simulink library "carnotUIBK"  (R2024b)
settings: Solver=VariableStepAuto  StartTime=0.0  StopTime=10.0  RelTol=1e-3  EnableMultiTasking=on
values from neighbouring files (symbols this model uses):
  area = area + room(kk).area    [THERMALZONE.m]
  boundary = BOUNDARY()    [BUILDING.m]
  building = obj    [BUILDING.m]
  C = zeros(1,length(d)+1)    [CONSTRUCTION.m]
  cp = str2num(value)    [CONSTRUCTION.m]
  pos = find(d_layer>0)    [CONSTRUCTION.m]
  rho = str2num(value)    [CONSTRUCTION.m]
  type = 1    [CONSTRUCTION.m]
  zone = obj.zone(ind)    [THERMALZONE.m]
undefined symbols (not defined in the file or in its folder): A, amb_factor, B, const, control, Dd, get_building, height, p, Qdot_C, Qdot_H, Qdot_I_electricity, Qdot_I_light, Qdot_I_person, Qdot_S, Qdot_T_ground, Qdot_T_neighbour, Qdot_T_opaque, Qdot_T_window, Qdot_V_infiltration, Qdot_V_mech, Qdot_V_window, r_frame, solar_ratio, solar_ratio1, solar_ratio2, Tc, Tr, Ts, Uvalue, view_factor, wall, wallsurface, window, window_height, window_heigth, window_width, windowsurface, x_CO2, x_H2O, x_VOC, z
libraries: carnot x105, $bdroot x22, simulink x18, simulink_extras x14
(part 9 of 13)

== system carnotUIBK/gain/People/W//ppl (activity)/LUT_Qdot_hum1 ==
  note: LATENT/HUMID HEAT POWER emitted from a person in a room
  activity : Inport
  Top : Inport  Port=2
  Look-Up Table Qdot_hum : Subsystem  mask(Lookup Table (2-D)){x=[10 12 14 16 18 20 22 23 24 25 26 28 30 32 34], y=[0 1 2 3 4], t=[20 20 20 55 100; 20 20 20 55 100; 20 20 20 55 100; 21 21 21 58 105; 23 23 23 65 115; 25 25 25 75 130; 30 30 30 85 145; 35 35 35 90 155; 40 40 40 95 160; 45 45 45 100 167; 50 50 50 105 175; 60 60 60 115 190; 70 70 70 125 205; 80 80 80 135 225; 90 90 90 145 245]}
      mask prompts: x "Row:"; y "Column:"; t "Table:"
      mask help: Performs 2-D linear interpolation of input values using the specified input/output table. Extrapolation is performed outside the table boundaries.
      mask init:
      | [r,c]=size(t);
      | x=reshape(x,prod(size(x)),1);
      | xi=x(:,ones(1,c));
      | minx=min(x); maxx=max(x);
      | mint=min(min(t)); maxt=max(max(t));
      mask Display: plot(xi,t,[minx maxx],[mint mint],[minx minx],[mint maxt])
  Qdot_hum : Outport  InitialOutput=0  VectorParamsAs1DForOutWhenUnconnected=off
  wires:
  Top/1 -> Look-Up Table Qdot_hum/1(Rows)
  activity/1 -> Look-Up Table Qdot_hum/2(Cols)
  Look-Up Table Qdot_hum/1(U) -> Qdot_hum/1

== system carnotUIBK/gain/People/W//ppl (activity)/LUT_mdot_CO2 ==
  note: CO2 MASS FLOW emitted from a person in a room
  activity : Inport
  Look-Up mdot_CO2 : Lookup  InputValues=[0 1 2 3 4]  Table=[0.567 0.708 1.133 2.031 3.305]*10^-5
  mdot_CO2 : Outport  InitialOutput=0  VectorParamsAs1DForOutWhenUnconnected=off
  wires:
  Look-Up mdot_CO2/1 -> mdot_CO2/1
  activity/1 -> Look-Up mdot_CO2/1

== system carnotUIBK/gain/People/W//ppl (activity)/LUT_mdot_H2O ==
  note: WATER MASS FLOW emitted from a person in a room
  activity : Inport
  Top : Inport  Port=2
  Look-Up Table mdot_H2O : Subsystem  mask(Lookup Table (2-D)){x=[10 12 14 16 18 20 22 23 24 25 26 32], y=[0 1 2 3 4], t=[30 30 30 90 150; 30 30 30 90 150; 30 30 30 90 150; 30 30 30 90 155; 35 35 35 95 165; 40 40 40 110 185; 45 45 45 125 200; 50 50 50 130 210; 55 55 55 130 225; 60 60 60 140 240; 65 65 65 150 270; 120 120 120 250 450]/(3.6*1e6)}
      mask prompts: x "Row:"; y "Column:"; t "Table:"
      mask help: Performs 2-D linear interpolation of input values using the specified input/output table. Extrapolation is performed outside the table boundaries.
      mask init:
      | [r,c]=size(t);
      | x=reshape(x,prod(size(x)),1);
      | xi=x(:,ones(1,c));
      | minx=min(x); maxx=max(x);
      | mint=min(min(t)); maxt=max(max(t));
      mask Display: plot(xi,t,[minx maxx],[mint mint],[minx minx],[mint maxt])
  mdot_H2O : Outport  InitialOutput=0  VectorParamsAs1DForOutWhenUnconnected=off
  wires:
  Look-Up Table mdot_H2O/1(U) -> mdot_H2O/1
  activity/1 -> Look-Up Table mdot_H2O/2(Cols)
  Top/1 -> Look-Up Table mdot_H2O/1(Rows)

== system carnotUIBK/gain/People/W//ppl (constant)/LUT_mdot_CO2 ==
  note: CO2 MASS FLOW emitted from a person in a room
  activity : Inport
  Look-Up mdot_CO2 : Lookup  InputValues=[0 1 2 3 4]  Table=[0.567 0.708 1.133 2.031 3.305]*10^-5
  mdot_CO2 : Outport  InitialOutput=0  VectorParamsAs1DForOutWhenUnconnected=off
  wires:
  Look-Up mdot_CO2/1 -> mdot_CO2/1
  activity/1 -> Look-Up mdot_CO2/1

== system carnotUIBK/gain/People/W//ppl (constant)/LUT_mdot_H2O ==
  note: WATER MASS FLOW emitted from a person in a room
  activity : Inport
  Top : Inport  Port=2
  Look-Up Table mdot_H2O : Subsystem  mask(Lookup Table (2-D)){x=[10 12 14 16 18 20 22 23 24 25 26 32], y=[0 1 2 3 4], t=[30 30 30 90 150; 30 30 30 90 150; 30 30 30 90 150; 30 30 30 90 155; 35 35 35 95 165; 40 40 40 110 185; 45 45 45 125 200; 50 50 50 130 210; 55 55 55 130 225; 60 60 60 140 240; 65 65 65 150 270; 120 120 120 250 450]/(3.6*1e6)}
      mask prompts: x "Row:"; y "Column:"; t "Table:"
      mask help: Performs 2-D linear interpolation of input values using the specified input/output table. Extrapolation is performed outside the table boundaries.
      mask init:
      | [r,c]=size(t);
      | x=reshape(x,prod(size(x)),1);
      | xi=x(:,ones(1,c));
      | minx=min(x); maxx=max(x);
      | mint=min(min(t)); maxt=max(max(t));
      mask Display: plot(xi,t,[minx maxx],[mint mint],[minx minx],[mint maxt])
  mdot_H2O : Outport  InitialOutput=0  VectorParamsAs1DForOutWhenUnconnected=off
  wires:
  Look-Up Table mdot_H2O/1(U) -> mdot_H2O/1
  activity/1 -> Look-Up Table mdot_H2O/2(Cols)
  Top/1 -> Look-Up Table mdot_H2O/1(Rows)

== system carnotUIBK/infiltration/infiltration_pressure/infiltration_pressure/dP_infiltration ==
  T_int : Inport
  T_ext : Inport  Port=2
  windspeed : Inport  Port=3
  wind_angle : Inport  Port=4
  air_density_ext : Inport  Port=5
  H_window : Inport  Port=6
  add_coeff_wind : Inport  Port=7
  facade_angle : Inport  Port=8
  Add : Sum
  Add1 : Sum
  Divide : Product  Inputs=/****
  Gain : Gain  Gain=0.5
  K : Constant  Value=273.15
  Product : Product
  Product1 : Product  Inputs=3
  Sum : Sum  Inputs=|+-
  calculate wind_coeff : Subsystem
  g : Constant  Value=9.81
  half of window height : Gain  Gain=0.5
  dP_total : Outport  VectorParamsAs1DForOutWhenUnconnected=off
  wires:
  T_int/1 -> Add1/2, Sum/1
  T_ext/1 -> Sum/2
  Sum/1 -> Divide/2  "delta_T"
  air_density_ext/1 -> Product1/1, Divide/4
  Product/1 -> Gain/1
  Gain/1 -> Product1/3
  Add/1 -> dP_total/1
  g/1 -> Divide/3
  half of window height/1 -> Divide/5
  H_window/1 -> half of window height/1
  wind_angle/1 -> calculate wind_coeff/1(wind_angle)
  calculate wind_coeff/1(wind_coeff) -> Product1/2
  add_coeff_wind/1 -> calculate wind_coeff/2(additional_coeff_wind)
  facade_angle/1 -> calculate wind_coeff/3(facade_angle)
  Product1/1 -> Add/2
  windspeed/1 -> Product/1, Product/2
  Divide/1 -> Add/1
  K/1 -> Add1/1
  Add1/1 -> Divide/1

== system carnotUIBK/infiltration/infiltration_pressure/infiltration_pressure/power_law_infiltration ==
  dP : Inport
  C : Inport  Port=2
  n : Inport  Port=3
  density : Inport  Port=4
  1/3600 : Gain  Gain=1/3600
  Product2 : Product
  Product4 : Product
  abs : Abs  SaturateOnIntegerOverflow=off
  pow_law : Math  Operator=pow  SignedPower=on
  m_dot : Outport  VectorParamsAs1DForOutWhenUnconnected=off
  wires:
  pow_law/1 -> Product2/1
  C/1 -> 1/3600/1
  Product2/1 -> Product4/1
  n/1 -> pow_law/2
  dP/1 -> abs/1
  density/1 -> Product4/2
  Product4/1 -> m_dot/1
  1/3600/1 -> Product2/2
  abs/1 -> pow_law/1

== system carnotUIBK/room_node/1-node/pressure/Subsystem ==
  note: (J/(kg*K)
  T : Inport
  Celsius2Kelvin : Bias  Bias=273.15  SaturateOnIntegerOverflow=off
  air_gas_constant : Gain  Gain=287  SaturateOnIntegerOverflow=on  OutDataTypeStr=Inherit: Same as input  ParamDataTypeStr=Inherit: Same as input
  R*T ' : Outport  VectorParamsAs1DForOutWhenUnconnected=off
  wires:
  Celsius2Kelvin/1 -> air_gas_constant/1
  T/1 -> Celsius2Kelvin/1
  air_gas_constant/1 -> R*T '/1

== system carnotUIBK/room_node/1-node/pressure/Transfer Fcn (with initial outputs)1 ==
  In1 : Inport
  State Space : StateSpace  A=A  B=B  C=C  D=Dd  InitialCondition=X0
  Out1 : Outport  InitialOutput=0  VectorParamsAs1DForOutWhenUnconnected=off
  wires:
  State Space/1 -> Out1/1
  In1/1 -> State Space/1

== system carnotUIBK/room_node/2-node/density and capacity/Transfer Fcn (with initial outputs) ==
  In1 : Inport
  State Space : StateSpace  A=A  B=B  C=C  D=Dd  InitialCondition=X0
  Out1 : Outport  InitialOutput=0  VectorParamsAs1DForOutWhenUnconnected=off
  wires:
  In1/1 -> State Space/1
  State Space/1 -> Out1/1

== system carnotUIBK/room_node/2-node/pressure/Subsystem ==
  note: (J/(kg*K)
  T : Inport
  Celsius2Kelvin : Bias  Bias=273.15  SaturateOnIntegerOverflow=off
  air_gas_constant : Gain  Gain=287  SaturateOnIntegerOverflow=on  OutDataTypeStr=Inherit: Same as input  ParamDataTypeStr=Inherit: Same as input
  R*T ' : Outport  VectorParamsAs1DForOutWhenUnconnected=off
  wires:
  Celsius2Kelvin/1 -> air_gas_constant/1
  T/1 -> Celsius2Kelvin/1
  air_gas_constant/1 -> R*T '/1

== system carnotUIBK/room_node/2-node/pressure/Transfer Fcn (with initial outputs)1 ==
  In1 : Inport
  State Space : StateSpace  A=A  B=B  C=C  D=Dd  InitialCondition=X0
  Out1 : Outport  InitialOutput=0  VectorParamsAs1DForOutWhenUnconnected=off
  wires:
  State Space/1 -> Out1/1
  In1/1 -> State Space/1

== system carnotUIBK/room_node/2-node_ideal/pressure/Subsystem ==
  note: (J/(kg*K)
  T : Inport
  Celsius2Kelvin : Bias  Bias=273.15  SaturateOnIntegerOverflow=off
  air_gas_constant : Gain  Gain=287  SaturateOnIntegerOverflow=on  OutDataTypeStr=Inherit: Same as input  ParamDataTypeStr=Inherit: Same as input
  R*T ' : Outport  VectorParamsAs1DForOutWhenUnconnected=off
  wires:
  Celsius2Kelvin/1 -> air_gas_constant/1
  T/1 -> Celsius2Kelvin/1
  air_gas_constant/1 -> R*T '/1

== system carnotUIBK/room_node/2-node_ideal/pressure/Transfer Fcn (with initial outputs)1 ==
  In1 : Inport
  State Space : StateSpace  A=A  B=B  C=C  D=Dd  InitialCondition=X0
  Out1 : Outport  InitialOutput=0  VectorParamsAs1DForOutWhenUnconnected=off
  wires:
  State Space/1 -> Out1/1
  In1/1 -> State Space/1

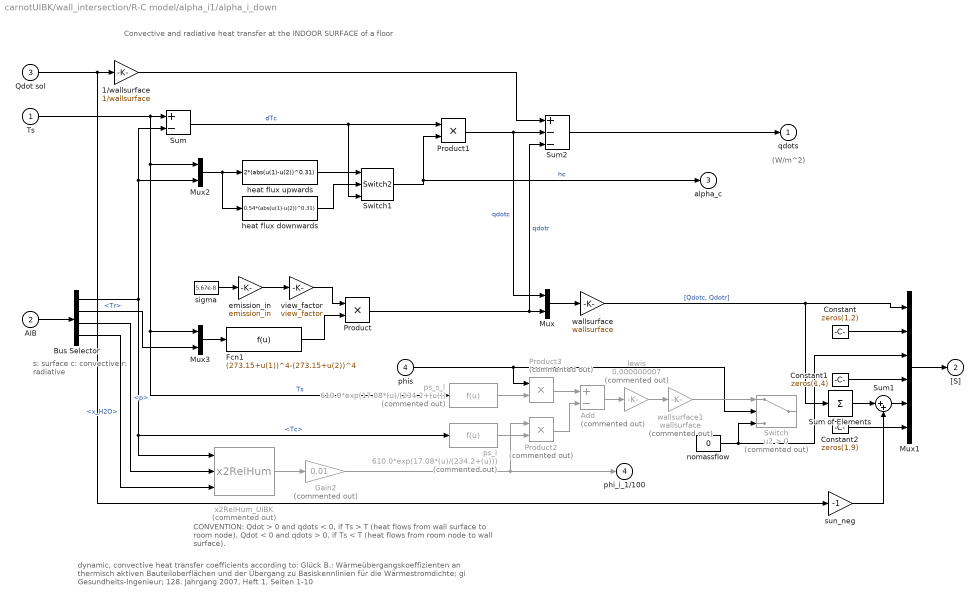
== system carnotUIBK/wall_intersection/R-C model/alpha_i1/alpha_i_down ==
  note: dynamic, convective heat transfer coefficients according to: Glück B.: Wärmeübergangskoeffizienten an thermisch aktiven Bauteiloberflächen
      | und der Übergang zu Basiskennlinien für die Wärmestromdichte; gi Gesundheits-Ingenieur; 128. Jahrgang 2007, Heft 1, Seiten 1-10
  note: s: surface
      | c: convective
      | r: radiative
  note: CONVENTION:
      | Qdot > 0 and qdots < 0, if Ts > T (heat flows from wall surface to room node),
      | Qdot < 0 and qdots > 0, if Ts < T (heat flows from room node to wall surface).
  note: Convective and radiative heat transfer at the INDOOR SURFACE of a floor
  note: (W/m^2)
  Ts : Inport
  AIB : Inport  Port=2
  Qdot sol : Inport  Port=3
  phis : Inport  Port=4
  1/wallsurface : Gain  Gain=1/wallsurface  SaturateOnIntegerOverflow=on  OutDataTypeStr=Inherit: Same as input  ParamDataTypeStr=Inherit: Same as input
  Add : Sum  Commented=on  Inputs=+-
  Bus Selector : BusSelector  OutputSignals=Tc,Tr,p,x_H2O
  Constant : Constant  Value=zeros(1,2)
  Constant1 : Constant  Value=zeros(1,4)
  Constant2 : Constant  Value=zeros(1,9)
  Fcn1 : Fcn  Expr=(273.15+u(1))^4-(273.15+u(2))^4
  Gain2 : Gain  Commented=on  Gain=0.01
  Mux : Mux  Inputs=2
  Mux1 : Mux  Inputs=[2 2 1 4 1 9]
  Mux2 : Mux  Inputs=2
  Mux3 : Mux  Inputs=2
  Product : Product  InputSameDT=on  RndMeth=Zero  SaturateOnIntegerOverflow=on  OutDataTypeStr=Inherit: Same as first input
  Product1 : Product  InputSameDT=on  RndMeth=Zero  SaturateOnIntegerOverflow=on  OutDataTypeStr=Inherit: Same as first input
  Product2 : Product  Commented=on  RndMeth=Zero
  Product3 : Product  Commented=on  RndMeth=Zero
  Sum : Sum  Inputs=+-  InputSameDT=on  SaturateOnIntegerOverflow=on  OutDataTypeStr=Inherit: Same as first input
  Sum of Elements : Sum  Inputs=+
  Sum1 : Sum  Inputs=|++
  Sum2 : Sum  Inputs=+--  InputSameDT=on  SaturateOnIntegerOverflow=on  OutDataTypeStr=Inherit: Same as first input
  Switch : Switch  Commented=on  Criteria=u2 > Threshold  SaturateOnIntegerOverflow=off  InputSameDT=off
  Switch1 : $bdroot/wall_intersection/R-C model/alpha_i1/alpha_i_up/Switch2  constCTR=0
  emission_in : Gain  Gain=emission_in  SaturateOnIntegerOverflow=on  OutDataTypeStr=Inherit: Same as input  ParamDataTypeStr=Inherit: Same as input
  heat flux downwards : Fcn  Expr=0.54*(abs(u(1)-u(2))^0.31)
  heat flux upwards : Fcn  Expr=2*(abs(u(1)-u(2))^0.31)
  lewis : Gain  Commented=on  Gain=0.000000007  SaturateOnIntegerOverflow=on  OutDataTypeStr=Inherit: Same as input  ParamDataTypeStr=Inherit: Same as input
  nomassflow : Constant  Value=0
  ps_l : Fcn  Commented=on  Expr=610.0*exp(17.08*(u)/(234.2+(u)))
  ps_s_l : Fcn  Commented=on  Expr=610.0*exp(17.08*(u)/(234.2+(u)))
  sigma : Constant  Value=5.67e-8
  sun_neg : Gain  Gain=-1  SaturateOnIntegerOverflow=on  OutDataTypeStr=Inherit: Same as input  ParamDataTypeStr=Inherit: Same as input
  view_factor : Gain  Gain=view_factor  SaturateOnIntegerOverflow=on  OutDataTypeStr=Inherit: Same as input  ParamDataTypeStr=Inherit: Same as input
  wallsurface : Gain  Gain=wallsurface  SaturateOnIntegerOverflow=on  OutDataTypeStr=Inherit: Same as input  ParamDataTypeStr=Inherit: Same as input
  wallsurface1 : Gain  Commented=on  Gain=wallsurface  SaturateOnIntegerOverflow=on  OutDataTypeStr=Inherit: Same as input  ParamDataTypeStr=Inherit: Same as input
  x2RelHum_UIBK : carnot/Basic/Material_Properties/x2RelHum  Commented=on
      settings: SourceProductName=Carnot
  qdots : Outport  InitialOutput=0  VectorParamsAs1DForOutWhenUnconnected=off
  "[S]" : Outport  Port=2  InitialOutput=0  VectorParamsAs1DForOutWhenUnconnected=off
  alpha_c : Outport  Port=3  InitialOutput=0  VectorParamsAs1DForOutWhenUnconnected=off
  phi_i_1/100 : Outport  Port=4  InitialOutput=0  VectorParamsAs1DForOutWhenUnconnected=off
  wires:
  heat flux downwards/1 -> Switch1/2
  heat flux upwards/1 -> Switch1/1
  Sum/1 -> Switch1/3, Product1/1  "dTc"
  1/wallsurface/1 -> Sum2/1
  wallsurface/1 -> Sum of Elements/1, Mux1/1  "[Qdotc, Qdotr]"
  Switch1/1 -> Product1/2, alpha_c/1  "hc"
  Product1/1 -> Sum2/2, Mux/1  "qdotc"
  Mux2/1 -> heat flux upwards/1, heat flux downwards/1
  Bus Selector/2 -> Mux3/2  "<Tr>"
  Ts/1 -> Mux2/1, Mux3/1, ps_s_l/1, Sum/1  "Ts"
  Mux/1 -> wallsurface/1
  Product/1 -> Mux/2, Sum2/3  "qdotr"
  emission_in/1 -> view_factor/1
  Bus Selector/1 -> x2RelHum_UIBK/1, ps_l/1, Mux2/2, Sum/2  "<Tc>"
  AIB/1 -> Bus Selector/1
  Sum2/1 -> qdots/1
  Mux1/1 -> "[S]"/1
  sigma/1 -> emission_in/1
  Mux3/1 -> Fcn1/1
  Fcn1/1 -> Product/2
  x2RelHum_UIBK/1 -> Gain2/1
  Bus Selector/3 -> x2RelHum_UIBK/2  "<p>"
  Bus Selector/4 -> x2RelHum_UIBK/3  "<x_H2O>"
  Gain2/1 -> phi_i_1/100/1, Product2/1
  lewis/1 -> wallsurface1/1
  Constant2/1 -> Mux1/6
  Constant1/1 -> Mux1/4
  Constant/1 -> Mux1/2
  ps_l/1 -> Product2/2
  ps_s_l/1 -> Product3/2
  Product3/1 -> Add/1
  Product2/1 -> Add/2
  Add/1 -> lewis/1
  phis/1 -> Switch/2, Product3/1
  view_factor/1 -> Product/1
  wallsurface1/1 -> Switch/1
  nomassflow/1 -> Mux1/3, Switch/3
  Sum1/1 -> Mux1/5
  Sum of Elements/1 -> Sum1/1
  Qdot sol/1 -> 1/wallsurface/1, sun_neg/1
  sun_neg/1 -> Sum1/2

== system carnotUIBK/wall_intersection/R-C model/alpha_i1/alpha_i_horizontal ==
  note: dynamic, convective heat transfer coefficients according to: Glück B.: Wärmeübergangskoeffizienten an thermisch aktiven Bauteiloberflächen
      | und der Übergang zu Basiskennlinien für die Wärmestromdichte; gi Gesundheits-Ingenieur; 128. Jahrgang 2007, Heft 1, Seiten 1-10
  note: s: surface
      | c: convective
      | r: radiative
  note: CONVENTION:
      | Qdot > 0 and qdots < 0, if Ts > T (heat flows from wall surface to room node),
      | Qdot < 0 and qdots > 0, if Ts < T (heat flows from room node to wall surface).
  note: Convective and radiative heat transfer at the INDOOR SURFACE of a VERTICAL OUTER WALL
  note: (W/m^2)
  Ts : Inport
  AIB : Inport  Port=2
  Qdot sol : Inport  Port=3
  phis : Inport  Port=4
  1/wallsurface : Gain  Gain=1/wallsurface  SaturateOnIntegerOverflow=on  OutDataTypeStr=Inherit: Same as input  ParamDataTypeStr=Inherit: Same as input
  Add : Sum  Commented=on  Inputs=+-
  Bus Selector : BusSelector  OutputSignals=Tc,Tr,p,x_H2O
  Constant : Constant  Value=zeros(1,2)
  Constant4 : Constant  Value=zeros(1,4)
  Constant5 : Constant  Value=zeros(1,9)
  Fcn : Fcn  Expr=1.6*(abs(u(1)-u(2)))^0.3
  Fcn1 : Fcn  Expr=(273.15+u(1))^4-(273.15+u(2))^4
  Gain2 : Gain  Commented=on  Gain=0.01
  Mux : Mux  Inputs=2
  Mux2 : Mux  Inputs=2
  Mux3 : Mux  Inputs=2
  Mux4 : Mux  Inputs=[2 2 1 4 1 9]
  Product : Product  InputSameDT=on  RndMeth=Zero  SaturateOnIntegerOverflow=on  OutDataTypeStr=Inherit: Same as first input
  Product1 : Product  InputSameDT=on  RndMeth=Zero  SaturateOnIntegerOverflow=on  OutDataTypeStr=Inherit: Same as first input
  Product2 : Product  Commented=on  RndMeth=Zero
  Product3 : Product  Commented=on  RndMeth=Zero
  Sum : Sum  Inputs=+-  InputSameDT=on  SaturateOnIntegerOverflow=on  OutDataTypeStr=Inherit: Same as first input
  Sum of Elements : Sum  Inputs=+
  Sum1 : Sum  Inputs=|++
  Sum2 : Sum  Inputs=+--  InputSameDT=on  SaturateOnIntegerOverflow=on  OutDataTypeStr=Inherit: Same as first input
  Switch : Switch  Commented=on  Criteria=u2 > Threshold  SaturateOnIntegerOverflow=off  InputSameDT=off
  emission_in : Gain  Gain=emission_in  SaturateOnIntegerOverflow=on  OutDataTypeStr=Inherit: Same as input  ParamDataTypeStr=Inherit: Same as input
  lewis : Gain  Commented=on  Gain=0.000000007  SaturateOnIntegerOverflow=on  OutDataTypeStr=Inherit: Same as input  ParamDataTypeStr=Inherit: Same as input
  nomassflow : Constant  Value=0
  ps_l : Fcn  Commented=on  Expr=610.0*exp(17.08*(u)/(234.2+(u)))
  ps_s_l : Fcn  Commented=on  Expr=610.0*exp(17.08*(u)/(234.2+(u)))
  sigma : Constant  Value=5.67e-8
  sun_neg : Gain  Gain=-1  SaturateOnIntegerOverflow=on  OutDataTypeStr=Inherit: Same as input  ParamDataTypeStr=Inherit: Same as input
  view_factor : Gain  Gain=view_factor  SaturateOnIntegerOverflow=on  OutDataTypeStr=Inherit: Same as input  ParamDataTypeStr=Inherit: Same as input
  wallsurface : Gain  Gain=wallsurface  SaturateOnIntegerOverflow=on  OutDataTypeStr=Inherit: Same as input  ParamDataTypeStr=Inherit: Same as input
  wallsurface1 : Gain  Commented=on  Gain=wallsurface  SaturateOnIntegerOverflow=on  OutDataTypeStr=Inherit: Same as input  ParamDataTypeStr=Inherit: Same as input
  x2RelHum_UIBK : carnot/Basic/Material_Properties/x2RelHum  Commented=on
      settings: SourceProductName=Carnot
  qdots : Outport  InitialOutput=0  VectorParamsAs1DForOutWhenUnconnected=off
  "[S]" : Outport  Port=2  InitialOutput=0  VectorParamsAs1DForOutWhenUnconnected=off
  alpha_c : Outport  Port=3  InitialOutput=0  VectorParamsAs1DForOutWhenUnconnected=off
  phi_i_1/100 : Outport  Port=4  InitialOutput=0  VectorParamsAs1DForOutWhenUnconnected=off
  wires:
  1/wallsurface/1 -> Sum2/1
  Qdot sol/1 -> sun_neg/1, 1/wallsurface/1
  wallsurface/1 -> Sum of Elements/1, Mux4/1  "[Qdotc, Qdotr]"
  Fcn/1 -> Product1/2, alpha_c/1  "hc"
  Product1/1 -> Sum2/2, Mux/1  "qdotc"
  Mux2/1 -> Fcn/1
  Bus Selector/2 -> Mux3/2  "<Tr>"
  Sum/1 -> Product1/1  "dTc"
  Ts/1 -> Mux2/1, Mux3/1, ps_s_l/1, Sum/1  "Ts"
  Mux/1 -> wallsurface/1
  Product/1 -> Mux/2, Sum2/3  "qdotr"
  emission_in/1 -> view_factor/1
  Bus Selector/1 -> x2RelHum_UIBK/1, ps_l/1, Mux2/2, Sum/2  "<Tc>"
  AIB/1 -> Bus Selector/1
  Sum2/1 -> qdots/1
  Mux4/1 -> "[S]"/1
  sigma/1 -> emission_in/1
  Mux3/1 -> Fcn1/1
  Fcn1/1 -> Product/2
  x2RelHum_UIBK/1 -> Gain2/1
  Bus Selector/3 -> x2RelHum_UIBK/2  "<p>"
  Bus Selector/4 -> x2RelHum_UIBK/3  "<x_H2O>"
  Gain2/1 -> phi_i_1/100/1, Product2/1
  lewis/1 -> wallsurface1/1
  ps_l/1 -> Product2/2
  ps_s_l/1 -> Product3/2
  Product3/1 -> Add/1
  Product2/1 -> Add/2
  Add/1 -> lewis/1
  phis/1 -> Switch/2, Product3/1
  view_factor/1 -> Product/1
  wallsurface1/1 -> Switch/1
  nomassflow/1 -> Mux4/3, Switch/3
  Constant/1 -> Mux4/2
  Constant5/1 -> Mux4/6
  Constant4/1 -> Mux4/4
  Sum1/1 -> Mux4/5
  Sum of Elements/1 -> Sum1/1
  sun_neg/1 -> Sum1/2

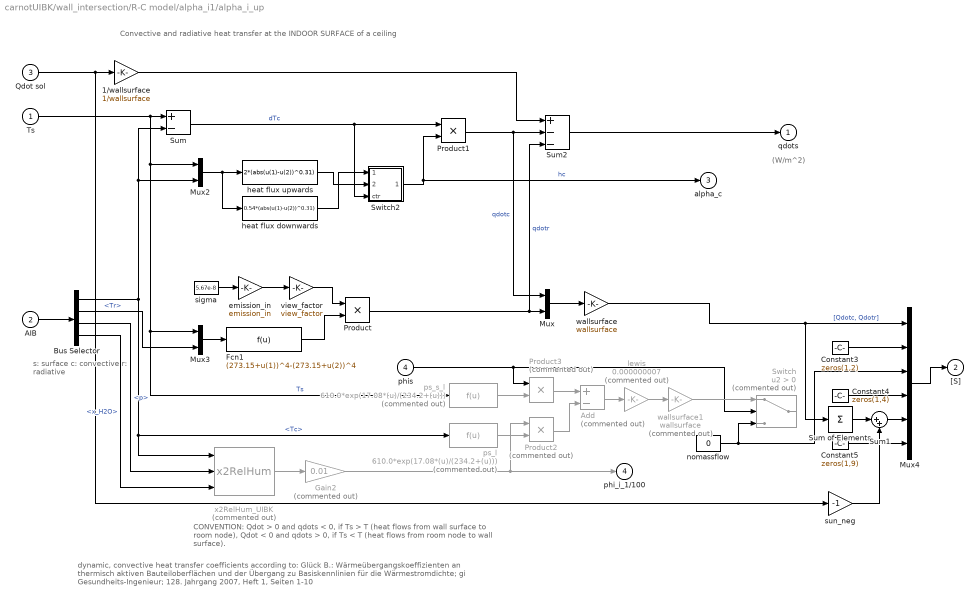
== system carnotUIBK/wall_intersection/R-C model/alpha_i1/alpha_i_up ==
  note: dynamic, convective heat transfer coefficients according to: Glück B.: Wärmeübergangskoeffizienten an thermisch aktiven Bauteiloberflächen
      | und der Übergang zu Basiskennlinien für die Wärmestromdichte; gi Gesundheits-Ingenieur; 128. Jahrgang 2007, Heft 1, Seiten 1-10
  note: s: surface
      | c: convective
      | r: radiative
  note: CONVENTION:
      | Qdot > 0 and qdots < 0, if Ts > T (heat flows from wall surface to room node),
      | Qdot < 0 and qdots > 0, if Ts < T (heat flows from room node to wall surface).
  note: Convective and radiative heat transfer at the INDOOR SURFACE of a ceiling
  note: (W/m^2)
  Ts : Inport
  AIB : Inport  Port=2
  Qdot sol : Inport  Port=3
  phis : Inport  Port=4
  1/wallsurface : Gain  Gain=1/wallsurface  SaturateOnIntegerOverflow=on  OutDataTypeStr=Inherit: Same as input  ParamDataTypeStr=Inherit: Same as input
  Add : Sum  Commented=on  Inputs=+-
  Bus Selector : BusSelector  OutputSignals=Tc,Tr,p,x_H2O
  Constant3 : Constant  Value=zeros(1,2)
  Constant4 : Constant  Value=zeros(1,4)
  Constant5 : Constant  Value=zeros(1,9)
  Fcn1 : Fcn  Expr=(273.15+u(1))^4-(273.15+u(2))^4
  Gain2 : Gain  Commented=on  Gain=0.01
  Mux : Mux  Inputs=2
  Mux2 : Mux  Inputs=2
  Mux3 : Mux  Inputs=2
  Mux4 : Mux  Inputs=[2 2 1 4 1 9]
  Product : Product  InputSameDT=on  RndMeth=Zero  SaturateOnIntegerOverflow=on  OutDataTypeStr=Inherit: Same as first input
  Product1 : Product  InputSameDT=on  RndMeth=Zero  SaturateOnIntegerOverflow=on  OutDataTypeStr=Inherit: Same as first input
  Product2 : Product  Commented=on  RndMeth=Zero
  Product3 : Product  Commented=on  RndMeth=Zero
  Sum : Sum  Inputs=+-  InputSameDT=on  SaturateOnIntegerOverflow=on  OutDataTypeStr=Inherit: Same as first input
  Sum of Elements : Sum  Inputs=+
  Sum1 : Sum  Inputs=|++
  Sum2 : Sum  Inputs=+--  InputSameDT=on  SaturateOnIntegerOverflow=on  OutDataTypeStr=Inherit: Same as first input
  Switch : Switch  Commented=on  Criteria=u2 > Threshold  SaturateOnIntegerOverflow=off  InputSameDT=off
  Switch2 : Subsystem  mask{constCTR=0}
      mask prompts: constCTR "Control threshold"
      mask DialogControl DescGroupVar Prompt: Switch
      mask DialogControl DescTextVar Prompt: If ctr signal > control threshold -> Out = Input 1; If ctr signal <= control threshold -> Out = Input 2
  emission_in : Gain  Gain=emission_in  SaturateOnIntegerOverflow=on  OutDataTypeStr=Inherit: Same as input  ParamDataTypeStr=Inherit: Same as input
  heat flux downwards : Fcn  Expr=0.54*(abs(u(1)-u(2))^0.31)
  heat flux upwards : Fcn  Expr=2*(abs(u(1)-u(2))^0.31)
  lewis : Gain  Commented=on  Gain=0.000000007  SaturateOnIntegerOverflow=on  OutDataTypeStr=Inherit: Same as input  ParamDataTypeStr=Inherit: Same as input
  nomassflow : Constant  Value=0
  ps_l : Fcn  Commented=on  Expr=610.0*exp(17.08*(u)/(234.2+(u)))
  ps_s_l : Fcn  Commented=on  Expr=610.0*exp(17.08*(u)/(234.2+(u)))
  sigma : Constant  Value=5.67e-8
  sun_neg : Gain  Gain=-1  SaturateOnIntegerOverflow=on  OutDataTypeStr=Inherit: Same as input  ParamDataTypeStr=Inherit: Same as input
  view_factor : Gain  Gain=view_factor  SaturateOnIntegerOverflow=on  OutDataTypeStr=Inherit: Same as input  ParamDataTypeStr=Inherit: Same as input
  wallsurface : Gain  Gain=wallsurface  SaturateOnIntegerOverflow=on  OutDataTypeStr=Inherit: Same as input  ParamDataTypeStr=Inherit: Same as input
  wallsurface1 : Gain  Commented=on  Gain=wallsurface  SaturateOnIntegerOverflow=on  OutDataTypeStr=Inherit: Same as input  ParamDataTypeStr=Inherit: Same as input
  x2RelHum_UIBK : carnot/Basic/Material_Properties/x2RelHum  Commented=on
      settings: SourceProductName=Carnot
  qdots : Outport  InitialOutput=0  VectorParamsAs1DForOutWhenUnconnected=off
  "[S]" : Outport  Port=2  InitialOutput=0  VectorParamsAs1DForOutWhenUnconnected=off
  alpha_c : Outport  Port=3  InitialOutput=0  VectorParamsAs1DForOutWhenUnconnected=off
  phi_i_1/100 : Outport  Port=4  InitialOutput=0  VectorParamsAs1DForOutWhenUnconnected=off
  wires:
  heat flux downwards/1 -> Switch2/1(Input1)
  heat flux upwards/1 -> Switch2/2(Input2)
  Sum/1 -> Switch2/3(ctr), Product1/1  "dTc"
  1/wallsurface/1 -> Sum2/1
  Qdot sol/1 -> sun_neg/1, 1/wallsurface/1
  Switch2/1(Out) -> alpha_c/1, Product1/2  "hc"
  Product1/1 -> Sum2/2, Mux/1  "qdotc"
  Mux2/1 -> heat flux upwards/1, heat flux downwards/1
  Bus Selector/2 -> Mux3/2  "<Tr>"
  Ts/1 -> Mux2/1, Mux3/1, ps_s_l/1, Sum/1  "Ts"
  Mux/1 -> wallsurface/1
  Product/1 -> Mux/2, Sum2/3  "qdotr"
  emission_in/1 -> view_factor/1
  Bus Selector/1 -> x2RelHum_UIBK/1, ps_l/1, Mux2/2, Sum/2  "<Tc>"
  AIB/1 -> Bus Selector/1
  Sum2/1 -> qdots/1
  sigma/1 -> emission_in/1
  Mux3/1 -> Fcn1/1
  Fcn1/1 -> Product/2
  x2RelHum_UIBK/1 -> Gain2/1
  Bus Selector/3 -> x2RelHum_UIBK/2  "<p>"
  Bus Selector/4 -> x2RelHum_UIBK/3  "<x_H2O>"
  Gain2/1 -> phi_i_1/100/1, Product2/1
  lewis/1 -> wallsurface1/1
  ps_l/1 -> Product2/2
  ps_s_l/1 -> Product3/2
  Product3/1 -> Add/1
  Product2/1 -> Add/2
  Add/1 -> lewis/1
  phis/1 -> Switch/2, Product3/1
  view_factor/1 -> Product/1
  wallsurface1/1 -> Switch/1
  nomassflow/1 -> Mux4/3, Switch/3
  wallsurface/1 -> Sum of Elements/1, Mux4/1  "[Qdotc, Qdotr]"
  Mux4/1 -> "[S]"/1
  Constant5/1 -> Mux4/6
  Constant4/1 -> Mux4/4
  Constant3/1 -> Mux4/2
  Sum of Elements/1 -> Sum1/1
  Sum1/1 -> Mux4/5
  sun_neg/1 -> Sum1/2

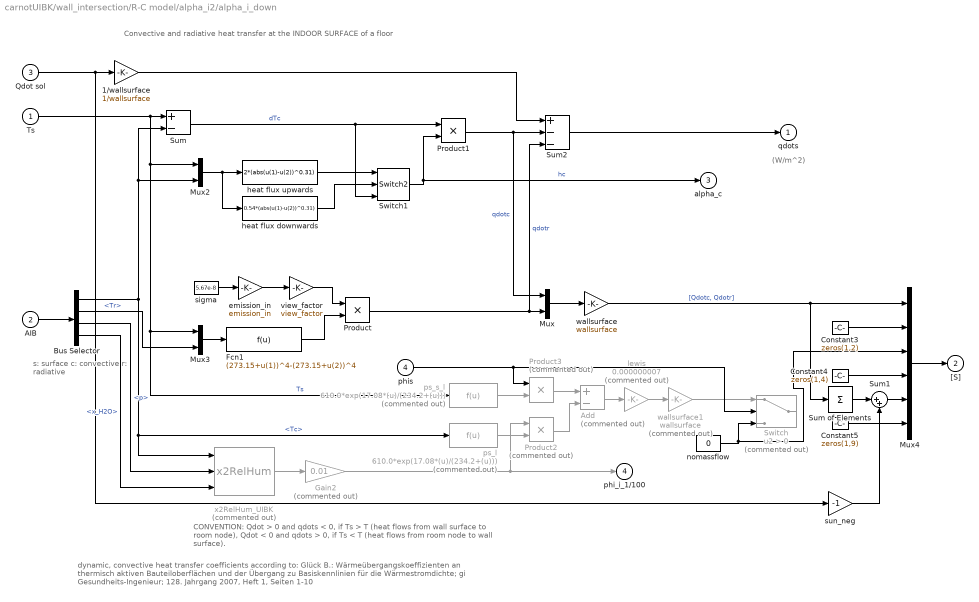
== system carnotUIBK/wall_intersection/R-C model/alpha_i2/alpha_i_down ==
  note: (W/m^2)
  note: Convective and radiative heat transfer at the INDOOR SURFACE of a floor
  note: CONVENTION:
      | Qdot > 0 and qdots < 0, if Ts > T (heat flows from wall surface to room node),
      | Qdot < 0 and qdots > 0, if Ts < T (heat flows from room node to wall surface).
  note: s: surface
      | c: convective
      | r: radiative
  note: dynamic, convective heat transfer coefficients according to: Glück B.: Wärmeübergangskoeffizienten an thermisch aktiven Bauteiloberflächen
      | und der Übergang zu Basiskennlinien für die Wärmestromdichte; gi Gesundheits-Ingenieur; 128. Jahrgang 2007, Heft 1, Seiten 1-10
  Ts : Inport
  AIB : Inport  Port=2
  Qdot sol : Inport  Port=3
  phis : Inport  Port=4
  1/wallsurface : Gain  Gain=1/wallsurface  SaturateOnIntegerOverflow=on  OutDataTypeStr=Inherit: Same as input  ParamDataTypeStr=Inherit: Same as input
  Add : Sum  Commented=on  Inputs=+-
  Bus Selector : BusSelector  OutputSignals=Tc,Tr,p,x_H2O
  Constant3 : Constant  Value=zeros(1,2)
  Constant4 : Constant  Value=zeros(1,4)
  Constant5 : Constant  Value=zeros(1,9)
  Fcn1 : Fcn  Expr=(273.15+u(1))^4-(273.15+u(2))^4
  Gain2 : Gain  Commented=on  Gain=0.01
  Mux : Mux  Inputs=2
  Mux2 : Mux  Inputs=2
  Mux3 : Mux  Inputs=2
  Mux4 : Mux  Inputs=[2 2 1 4 1 9]
  Product : Product  InputSameDT=on  RndMeth=Zero  SaturateOnIntegerOverflow=on  OutDataTypeStr=Inherit: Same as first input
  Product1 : Product  InputSameDT=on  RndMeth=Zero  SaturateOnIntegerOverflow=on  OutDataTypeStr=Inherit: Same as first input
  Product2 : Product  Commented=on  RndMeth=Zero
  Product3 : Product  Commented=on  RndMeth=Zero
  Sum : Sum  Inputs=+-  InputSameDT=on  SaturateOnIntegerOverflow=on  OutDataTypeStr=Inherit: Same as first input
  Sum of Elements : Sum  Inputs=+
  Sum1 : Sum  Inputs=|++
  Sum2 : Sum  Inputs=+--  InputSameDT=on  SaturateOnIntegerOverflow=on  OutDataTypeStr=Inherit: Same as first input
  Switch : Switch  Commented=on  Criteria=u2 > Threshold  SaturateOnIntegerOverflow=off  InputSameDT=off
  Switch1 : $bdroot/wall_intersection/R-C model/alpha_i1/alpha_i_up/Switch2  constCTR=0
  emission_in : Gain  Gain=emission_in  SaturateOnIntegerOverflow=on  OutDataTypeStr=Inherit: Same as input  ParamDataTypeStr=Inherit: Same as input
  heat flux downwards : Fcn  Expr=0.54*(abs(u(1)-u(2))^0.31)
  heat flux upwards : Fcn  Expr=2*(abs(u(1)-u(2))^0.31)
  lewis : Gain  Commented=on  Gain=0.000000007  SaturateOnIntegerOverflow=on  OutDataTypeStr=Inherit: Same as input  ParamDataTypeStr=Inherit: Same as input
  nomassflow : Constant  Value=0
  ps_l : Fcn  Commented=on  Expr=610.0*exp(17.08*(u)/(234.2+(u)))
  ps_s_l : Fcn  Commented=on  Expr=610.0*exp(17.08*(u)/(234.2+(u)))
  sigma : Constant  Value=5.67e-8
  sun_neg : Gain  Gain=-1  SaturateOnIntegerOverflow=on  OutDataTypeStr=Inherit: Same as input  ParamDataTypeStr=Inherit: Same as input
  view_factor : Gain  Gain=view_factor  SaturateOnIntegerOverflow=on  OutDataTypeStr=Inherit: Same as input  ParamDataTypeStr=Inherit: Same as input
  wallsurface : Gain  Gain=wallsurface  SaturateOnIntegerOverflow=on  OutDataTypeStr=Inherit: Same as input  ParamDataTypeStr=Inherit: Same as input
  wallsurface1 : Gain  Commented=on  Gain=wallsurface  SaturateOnIntegerOverflow=on  OutDataTypeStr=Inherit: Same as input  ParamDataTypeStr=Inherit: Same as input
  x2RelHum_UIBK : carnot/Basic/Material_Properties/x2RelHum  Commented=on
      settings: SourceProductName=Carnot
  qdots : Outport  InitialOutput=0  VectorParamsAs1DForOutWhenUnconnected=off
  "[S]" : Outport  Port=2  InitialOutput=0  VectorParamsAs1DForOutWhenUnconnected=off
  alpha_c : Outport  Port=3  InitialOutput=0  VectorParamsAs1DForOutWhenUnconnected=off
  phi_i_1/100 : Outport  Port=4  InitialOutput=0  VectorParamsAs1DForOutWhenUnconnected=off
  wires:
  nomassflow/1 -> Mux4/3, Switch/3
  wallsurface1/1 -> Switch/1
  view_factor/1 -> Product/1
  phis/1 -> Product3/1, Switch/2
  Add/1 -> lewis/1
  Product2/1 -> Add/2
  Product3/1 -> Add/1
  ps_s_l/1 -> Product3/2
  ps_l/1 -> Product2/2
  lewis/1 -> wallsurface1/1
  Gain2/1 -> Product2/1, phi_i_1/100/1
  Bus Selector/4 -> x2RelHum_UIBK/3  "<x_H2O>"
  Bus Selector/3 -> x2RelHum_UIBK/2  "<p>"
  x2RelHum_UIBK/1 -> Gain2/1
  Fcn1/1 -> Product/2
  Mux3/1 -> Fcn1/1
  sigma/1 -> emission_in/1
  Mux4/1 -> "[S]"/1
  Sum2/1 -> qdots/1
  AIB/1 -> Bus Selector/1
  Bus Selector/1 -> Sum/2, Mux2/2, x2RelHum_UIBK/1, ps_l/1  "<Tc>"
  emission_in/1 -> view_factor/1
  Product/1 -> Sum2/3, Mux/2  "qdotr"
  Mux/1 -> wallsurface/1
  Ts/1 -> Sum/1, ps_s_l/1, Mux3/1, Mux2/1  "Ts"
  Bus Selector/2 -> Mux3/2  "<Tr>"
  Mux2/1 -> heat flux downwards/1, heat flux upwards/1
  Product1/1 -> Mux/1, Sum2/2  "qdotc"
  Switch1/1 -> Product1/2, alpha_c/1  "hc"
  wallsurface/1 -> Sum of Elements/1, Mux4/1  "[Qdotc, Qdotr]"
  Qdot sol/1 -> sun_neg/1, 1/wallsurface/1
  1/wallsurface/1 -> Sum2/1
  Sum/1 -> Switch1/3, Product1/1  "dTc"
  heat flux upwards/1 -> Switch1/1
  heat flux downwards/1 -> Switch1/2
  Constant5/1 -> Mux4/6
  Constant4/1 -> Mux4/4
  Constant3/1 -> Mux4/2
  Sum of Elements/1 -> Sum1/1
  Sum1/1 -> Mux4/5
  sun_neg/1 -> Sum1/2

== system carnotUIBK/wall_intersection/R-C model/alpha_i2/alpha_i_horizontal ==
  note: (W/m^2)
  note: Convective and radiative heat transfer at the INDOOR SURFACE of a VERTICAL OUTER WALL
  note: CONVENTION:
      | Qdot > 0 and qdots < 0, if Ts > T (heat flows from wall surface to room node),
      | Qdot < 0 and qdots > 0, if Ts < T (heat flows from room node to wall surface).
  note: s: surface
      | c: convective
      | r: radiative
  note: dynamic, convective heat transfer coefficients according to: Glück B.: Wärmeübergangskoeffizienten an thermisch aktiven Bauteiloberflächen
      | und der Übergang zu Basiskennlinien für die Wärmestromdichte; gi Gesundheits-Ingenieur; 128. Jahrgang 2007, Heft 1, Seiten 1-10
  Ts : Inport
  AIB : Inport  Port=2
  Qdot sol : Inport  Port=3
  phis : Inport  Port=4
  1/wallsurface : Gain  Gain=1/wallsurface  SaturateOnIntegerOverflow=on  OutDataTypeStr=Inherit: Same as input  ParamDataTypeStr=Inherit: Same as input
  Add : Sum  Commented=on  Inputs=+-
  Bus Selector : BusSelector  OutputSignals=Tc,Tr,p,x_H2O
  Constant3 : Constant  Value=zeros(1,2)
  Constant4 : Constant  Value=zeros(1,4)
  Constant5 : Constant  Value=zeros(1,9)
  Fcn : Fcn  Expr=1.6*(abs(u(1)-u(2)))^0.3
  Fcn1 : Fcn  Expr=(273.15+u(1))^4-(273.15+u(2))^4
  Gain2 : Gain  Commented=on  Gain=0.01
  Mux : Mux  Inputs=2
  Mux2 : Mux  Inputs=2
  Mux3 : Mux  Inputs=2
  Mux4 : Mux  Inputs=[2 2 1 4 1 9]
  Product : Product  InputSameDT=on  RndMeth=Zero  SaturateOnIntegerOverflow=on  OutDataTypeStr=Inherit: Same as first input
  Product1 : Product  InputSameDT=on  RndMeth=Zero  SaturateOnIntegerOverflow=on  OutDataTypeStr=Inherit: Same as first input
  Product2 : Product  Commented=on  RndMeth=Zero
  Product3 : Product  Commented=on  RndMeth=Zero
  Sum : Sum  Inputs=+-  InputSameDT=on  SaturateOnIntegerOverflow=on  OutDataTypeStr=Inherit: Same as first input
  Sum of Elements : Sum  Inputs=+
  Sum1 : Sum  Inputs=|++
  Sum2 : Sum  Inputs=+--  InputSameDT=on  SaturateOnIntegerOverflow=on  OutDataTypeStr=Inherit: Same as first input
  Switch : Switch  Commented=on  Criteria=u2 > Threshold  SaturateOnIntegerOverflow=off  InputSameDT=off
  emission_in : Gain  Gain=emission_in  SaturateOnIntegerOverflow=on  OutDataTypeStr=Inherit: Same as input  ParamDataTypeStr=Inherit: Same as input
  lewis : Gain  Commented=on  Gain=0.000000007  SaturateOnIntegerOverflow=on  OutDataTypeStr=Inherit: Same as input  ParamDataTypeStr=Inherit: Same as input
  nomassflow : Constant  Value=0
  ps_l : Fcn  Commented=on  Expr=610.0*exp(17.08*(u)/(234.2+(u)))
  ps_s_l : Fcn  Commented=on  Expr=610.0*exp(17.08*(u)/(234.2+(u)))
  sigma : Constant  Value=5.67e-8
  sun_neg : Gain  Gain=-1  SaturateOnIntegerOverflow=on  OutDataTypeStr=Inherit: Same as input  ParamDataTypeStr=Inherit: Same as input
  view_factor : Gain  Gain=view_factor  SaturateOnIntegerOverflow=on  OutDataTypeStr=Inherit: Same as input  ParamDataTypeStr=Inherit: Same as input
  wallsurface : Gain  Gain=wallsurface  SaturateOnIntegerOverflow=on  OutDataTypeStr=Inherit: Same as input  ParamDataTypeStr=Inherit: Same as input
  wallsurface1 : Gain  Commented=on  Gain=wallsurface  SaturateOnIntegerOverflow=on  OutDataTypeStr=Inherit: Same as input  ParamDataTypeStr=Inherit: Same as input
  x2RelHum_UIBK : carnot/Basic/Material_Properties/x2RelHum  Commented=on
      settings: SourceProductName=Carnot
  qdots : Outport  InitialOutput=0  VectorParamsAs1DForOutWhenUnconnected=off
  "[S]" : Outport  Port=2  InitialOutput=0  VectorParamsAs1DForOutWhenUnconnected=off
  alpha_c : Outport  Port=3  InitialOutput=0  VectorParamsAs1DForOutWhenUnconnected=off
  phi_i_1/100 : Outport  Port=4  InitialOutput=0  VectorParamsAs1DForOutWhenUnconnected=off
  wires:
  nomassflow/1 -> Mux4/3, Switch/3
  wallsurface1/1 -> Switch/1
  view_factor/1 -> Product/1
  phis/1 -> Product3/1, Switch/2
  Add/1 -> lewis/1
  Product2/1 -> Add/2
  Product3/1 -> Add/1
  ps_s_l/1 -> Product3/2
  ps_l/1 -> Product2/2
  lewis/1 -> wallsurface1/1
  Gain2/1 -> Product2/1, phi_i_1/100/1
  Bus Selector/4 -> x2RelHum_UIBK/3  "<x_H2O>"
  Bus Selector/3 -> x2RelHum_UIBK/2  "<p>"
  x2RelHum_UIBK/1 -> Gain2/1
  Fcn1/1 -> Product/2
  Mux3/1 -> Fcn1/1
  sigma/1 -> emission_in/1
  Mux4/1 -> "[S]"/1
  Sum2/1 -> qdots/1
  AIB/1 -> Bus Selector/1
  Bus Selector/1 -> Sum/2, Mux2/2, x2RelHum_UIBK/1, ps_l/1  "<Tc>"
  emission_in/1 -> view_factor/1
  Product/1 -> Sum2/3, Mux/2  "qdotr"
  Mux/1 -> wallsurface/1
  Ts/1 -> Sum/1, ps_s_l/1, Mux3/1, Mux2/1  "Ts"
  Sum/1 -> Product1/1  "dTc"
  Bus Selector/2 -> Mux3/2  "<Tr>"
  Mux2/1 -> Fcn/1
  Product1/1 -> Mux/1, Sum2/2  "qdotc"
  Fcn/1 -> alpha_c/1, Product1/2  "hc"
  wallsurface/1 -> Sum of Elements/1, Mux4/1  "[Qdotc, Qdotr]"
  Qdot sol/1 -> sun_neg/1, 1/wallsurface/1
  1/wallsurface/1 -> Sum2/1
  Constant5/1 -> Mux4/6
  Constant4/1 -> Mux4/4
  Constant3/1 -> Mux4/2
  Sum of Elements/1 -> Sum1/1
  Sum1/1 -> Mux4/5
  sun_neg/1 -> Sum1/2

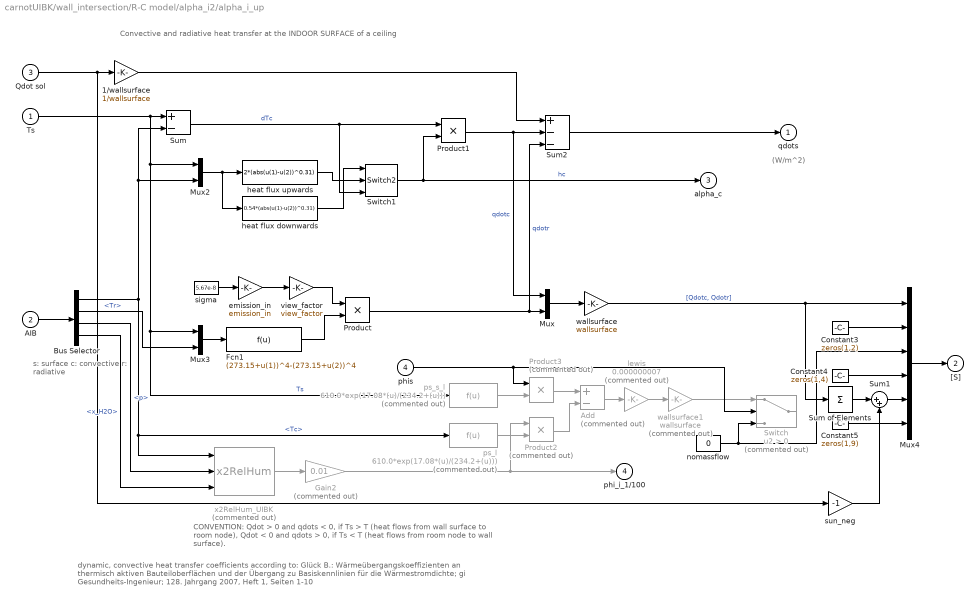
== system carnotUIBK/wall_intersection/R-C model/alpha_i2/alpha_i_up ==
  note: (W/m^2)
  note: Convective and radiative heat transfer at the INDOOR SURFACE of a ceiling
  note: CONVENTION:
      | Qdot > 0 and qdots < 0, if Ts > T (heat flows from wall surface to room node),
      | Qdot < 0 and qdots > 0, if Ts < T (heat flows from room node to wall surface).
  note: s: surface
      | c: convective
      | r: radiative
  note: dynamic, convective heat transfer coefficients according to: Glück B.: Wärmeübergangskoeffizienten an thermisch aktiven Bauteiloberflächen
      | und der Übergang zu Basiskennlinien für die Wärmestromdichte; gi Gesundheits-Ingenieur; 128. Jahrgang 2007, Heft 1, Seiten 1-10
  Ts : Inport
  AIB : Inport  Port=2
  Qdot sol : Inport  Port=3
  phis : Inport  Port=4
  1/wallsurface : Gain  Gain=1/wallsurface  SaturateOnIntegerOverflow=on  OutDataTypeStr=Inherit: Same as input  ParamDataTypeStr=Inherit: Same as input
  Add : Sum  Commented=on  Inputs=+-
  Bus Selector : BusSelector  OutputSignals=Tc,Tr,p,x_H2O
  Constant3 : Constant  Value=zeros(1,2)
  Constant4 : Constant  Value=zeros(1,4)
  Constant5 : Constant  Value=zeros(1,9)
  Fcn1 : Fcn  Expr=(273.15+u(1))^4-(273.15+u(2))^4
  Gain2 : Gain  Commented=on  Gain=0.01
  Mux : Mux  Inputs=2
  Mux2 : Mux  Inputs=2
  Mux3 : Mux  Inputs=2
  Mux4 : Mux  Inputs=[2 2 1 4 1 9]
  Product : Product  InputSameDT=on  RndMeth=Zero  SaturateOnIntegerOverflow=on  OutDataTypeStr=Inherit: Same as first input
  Product1 : Product  InputSameDT=on  RndMeth=Zero  SaturateOnIntegerOverflow=on  OutDataTypeStr=Inherit: Same as first input
  Product2 : Product  Commented=on  RndMeth=Zero
  Product3 : Product  Commented=on  RndMeth=Zero
  Sum : Sum  Inputs=+-  InputSameDT=on  SaturateOnIntegerOverflow=on  OutDataTypeStr=Inherit: Same as first input
  Sum of Elements : Sum  Inputs=+
  Sum1 : Sum  Inputs=|++
  Sum2 : Sum  Inputs=+--  InputSameDT=on  SaturateOnIntegerOverflow=on  OutDataTypeStr=Inherit: Same as first input
  Switch : Switch  Commented=on  Criteria=u2 > Threshold  SaturateOnIntegerOverflow=off  InputSameDT=off
  Switch1 : $bdroot/wall_intersection/R-C model/alpha_i1/alpha_i_up/Switch2  constCTR=0
  emission_in : Gain  Gain=emission_in  SaturateOnIntegerOverflow=on  OutDataTypeStr=Inherit: Same as input  ParamDataTypeStr=Inherit: Same as input
  heat flux downwards : Fcn  Expr=0.54*(abs(u(1)-u(2))^0.31)
  heat flux upwards : Fcn  Expr=2*(abs(u(1)-u(2))^0.31)
  lewis : Gain  Commented=on  Gain=0.000000007  SaturateOnIntegerOverflow=on  OutDataTypeStr=Inherit: Same as input  ParamDataTypeStr=Inherit: Same as input
  nomassflow : Constant  Value=0
  ps_l : Fcn  Commented=on  Expr=610.0*exp(17.08*(u)/(234.2+(u)))
  ps_s_l : Fcn  Commented=on  Expr=610.0*exp(17.08*(u)/(234.2+(u)))
  sigma : Constant  Value=5.67e-8
  sun_neg : Gain  Gain=-1  SaturateOnIntegerOverflow=on  OutDataTypeStr=Inherit: Same as input  ParamDataTypeStr=Inherit: Same as input
  view_factor : Gain  Gain=view_factor  SaturateOnIntegerOverflow=on  OutDataTypeStr=Inherit: Same as input  ParamDataTypeStr=Inherit: Same as input
  wallsurface : Gain  Gain=wallsurface  SaturateOnIntegerOverflow=on  OutDataTypeStr=Inherit: Same as input  ParamDataTypeStr=Inherit: Same as input
  wallsurface1 : Gain  Commented=on  Gain=wallsurface  SaturateOnIntegerOverflow=on  OutDataTypeStr=Inherit: Same as input  ParamDataTypeStr=Inherit: Same as input
  x2RelHum_UIBK : carnot/Basic/Material_Properties/x2RelHum  Commented=on
      settings: SourceProductName=Carnot
  qdots : Outport  InitialOutput=0  VectorParamsAs1DForOutWhenUnconnected=off
  "[S]" : Outport  Port=2  InitialOutput=0  VectorParamsAs1DForOutWhenUnconnected=off
  alpha_c : Outport  Port=3  InitialOutput=0  VectorParamsAs1DForOutWhenUnconnected=off
  phi_i_1/100 : Outport  Port=4  InitialOutput=0  VectorParamsAs1DForOutWhenUnconnected=off
  wires:
  nomassflow/1 -> Mux4/3, Switch/3
  wallsurface1/1 -> Switch/1
  view_factor/1 -> Product/1
  phis/1 -> Product3/1, Switch/2
  Add/1 -> lewis/1
  Product2/1 -> Add/2
  Product3/1 -> Add/1
  ps_s_l/1 -> Product3/2
  ps_l/1 -> Product2/2
  lewis/1 -> wallsurface1/1
  Gain2/1 -> Product2/1, phi_i_1/100/1
  Bus Selector/4 -> x2RelHum_UIBK/3  "<x_H2O>"
  Bus Selector/3 -> x2RelHum_UIBK/2  "<p>"
  x2RelHum_UIBK/1 -> Gain2/1
  Fcn1/1 -> Product/2
  Mux3/1 -> Fcn1/1
  sigma/1 -> emission_in/1
  Mux4/1 -> "[S]"/1
  Sum2/1 -> qdots/1
  AIB/1 -> Bus Selector/1
  Bus Selector/1 -> Sum/2, Mux2/2, x2RelHum_UIBK/1, ps_l/1  "<Tc>"
  emission_in/1 -> view_factor/1
  Product/1 -> Sum2/3, Mux/2  "qdotr"
  Mux/1 -> wallsurface/1
  Ts/1 -> Sum/1, ps_s_l/1, Mux3/1, Mux2/1  "Ts"
  Bus Selector/2 -> Mux3/2  "<Tr>"
  Mux2/1 -> heat flux downwards/1, heat flux upwards/1
  Product1/1 -> Mux/1, Sum2/2  "qdotc"
  Switch1/1 -> Product1/2, alpha_c/1  "hc"
  wallsurface/1 -> Sum of Elements/1, Mux4/1  "[Qdotc, Qdotr]"
  Qdot sol/1 -> sun_neg/1, 1/wallsurface/1
  1/wallsurface/1 -> Sum2/1
  Sum/1 -> Switch1/3, Product1/1  "dTc"
  heat flux upwards/1 -> Switch1/2
  heat flux downwards/1 -> Switch1/1
  Constant5/1 -> Mux4/6
  Constant4/1 -> Mux4/4
  Constant3/1 -> Mux4/2
  Sum of Elements/1 -> Sum1/1
  Sum1/1 -> Mux4/5
  sun_neg/1 -> Sum1/2

== system carnotUIBK/wall_intersection/UA/Rsi/down ==
  0.17+0.10 : Constant  Value=0.27
  Rsi : Outport  VectorParamsAs1DForOutWhenUnconnected=off
  wires:
  0.17+0.10/1 -> Rsi/1

== system carnotUIBK/wall_intersection/UA/Rsi/horizontal ==
  2x0.13 : Constant  Value=0.26
  Rsi : Outport  VectorParamsAs1DForOutWhenUnconnected=off
  wires:
  2x0.13/1 -> Rsi/1

== system carnotUIBK/wall_intersection/UA/Rsi/up ==
  0.10+0.17 : Constant  Value=0.27
  Rsi : Outport  VectorParamsAs1DForOutWhenUnconnected=off
  wires:
  0.10+0.17/1 -> Rsi/1

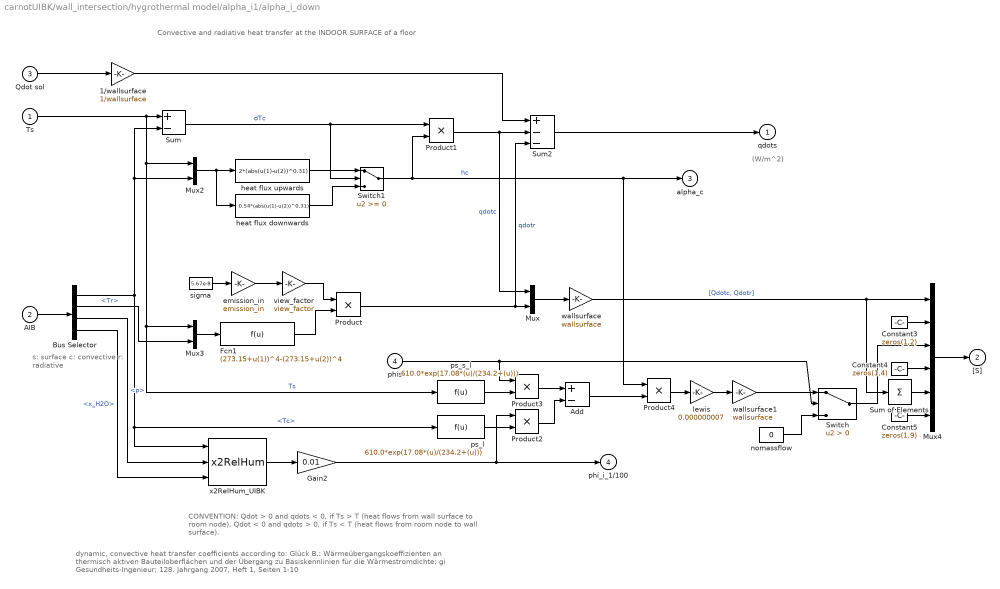
== system carnotUIBK/wall_intersection/hygrothermal model/alpha_i1/alpha_i_down ==
  note: dynamic, convective heat transfer coefficients according to: Glück B.: Wärmeübergangskoeffizienten an thermisch aktiven Bauteiloberflächen
      | und der Übergang zu Basiskennlinien für die Wärmestromdichte; gi Gesundheits-Ingenieur; 128. Jahrgang 2007, Heft 1, Seiten 1-10
  note: s: surface
      | c: convective
      | r: radiative
  note: CONVENTION:
      | Qdot > 0 and qdots < 0, if Ts > T (heat flows from wall surface to room node),
      | Qdot < 0 and qdots > 0, if Ts < T (heat flows from room node to wall surface).
  note: Convective and radiative heat transfer at the INDOOR SURFACE of a floor
  note: (W/m^2)
  Ts : Inport
  AIB : Inport  Port=2
  Qdot sol : Inport  Port=3
  phis : Inport  Port=4
  1/wallsurface : Gain  Gain=1/wallsurface  SaturateOnIntegerOverflow=on  OutDataTypeStr=Inherit: Same as input  ParamDataTypeStr=Inherit: Same as input
  Add : Sum  Inputs=+-
  Bus Selector : BusSelector  OutputSignals=Tc,Tr,p,x_H2O
  Constant3 : Constant  Value=zeros(1,2)
  Constant4 : Constant  Value=zeros(1,4)
  Constant5 : Constant  Value=zeros(1,9)
  Fcn1 : Fcn  Expr=(273.15+u(1))^4-(273.15+u(2))^4
  Gain2 : Gain  Gain=0.01
  Mux : Mux  Inputs=2
  Mux2 : Mux  Inputs=2
  Mux3 : Mux  Inputs=2
  Mux4 : Mux  Inputs=[2 2 1 4 1 9]
  Product : Product  InputSameDT=on  RndMeth=Zero  SaturateOnIntegerOverflow=on  OutDataTypeStr=Inherit: Same as first input
  Product1 : Product  InputSameDT=on  RndMeth=Zero  SaturateOnIntegerOverflow=on  OutDataTypeStr=Inherit: Same as first input
  Product2 : Product  RndMeth=Zero
  Product3 : Product  RndMeth=Zero
  Product4 : Product  InputSameDT=on  RndMeth=Zero  SaturateOnIntegerOverflow=on  OutDataTypeStr=Inherit: Same as first input
  Sum : Sum  Inputs=+-  InputSameDT=on  SaturateOnIntegerOverflow=on  OutDataTypeStr=Inherit: Same as first input
  Sum of Elements : Sum  Inputs=+
  Sum2 : Sum  Inputs=+--  InputSameDT=on  SaturateOnIntegerOverflow=on  OutDataTypeStr=Inherit: Same as first input
  Switch : Switch  Criteria=u2 > Threshold  SaturateOnIntegerOverflow=off  InputSameDT=off
  Switch1 : Switch  SaturateOnIntegerOverflow=off  InputSameDT=off
  emission_in : Gain  Gain=emission_in  SaturateOnIntegerOverflow=on  OutDataTypeStr=Inherit: Same as input  ParamDataTypeStr=Inherit: Same as input
  heat flux downwards : Fcn  Expr=0.54*(abs(u(1)-u(2))^0.31)
  heat flux upwards : Fcn  Expr=2*(abs(u(1)-u(2))^0.31)
  lewis : Gain  Gain=0.000000007  SaturateOnIntegerOverflow=on  OutDataTypeStr=Inherit: Same as input  ParamDataTypeStr=Inherit: Same as input
  nomassflow : Constant  Value=0
  ps_l : Fcn  Expr=610.0*exp(17.08*(u)/(234.2+(u)))
  ps_s_l : Fcn  Expr=610.0*exp(17.08*(u)/(234.2+(u)))
  sigma : Constant  Value=5.67e-8
  view_factor : Gain  Gain=view_factor  SaturateOnIntegerOverflow=on  OutDataTypeStr=Inherit: Same as input  ParamDataTypeStr=Inherit: Same as input
  wallsurface : Gain  Gain=wallsurface  SaturateOnIntegerOverflow=on  OutDataTypeStr=Inherit: Same as input  ParamDataTypeStr=Inherit: Same as input
  wallsurface1 : Gain  Gain=wallsurface  SaturateOnIntegerOverflow=on  OutDataTypeStr=Inherit: Same as input  ParamDataTypeStr=Inherit: Same as input
  x2RelHum_UIBK : carnot/Basic/Material_Properties/x2RelHum
      settings: SourceProductName=Carnot
  qdots : Outport  InitialOutput=0  VectorParamsAs1DForOutWhenUnconnected=off
  "[S]" : Outport  Port=2  InitialOutput=0  VectorParamsAs1DForOutWhenUnconnected=off
  alpha_c : Outport  Port=3  InitialOutput=0  VectorParamsAs1DForOutWhenUnconnected=off
  phi_i_1/100 : Outport  Port=4  InitialOutput=0  VectorParamsAs1DForOutWhenUnconnected=off
  wires:
  heat flux downwards/1 -> Switch1/3
  heat flux upwards/1 -> Switch1/1
  Sum/1 -> Product1/1, Switch1/2  "dTc"
  1/wallsurface/1 -> Sum2/1
  Qdot sol/1 -> 1/wallsurface/1
  wallsurface/1 -> Sum of Elements/1, Mux4/1  "[Qdotc, Qdotr]"
  Switch1/1 -> Product4/1, alpha_c/1, Product1/2  "hc"
  Product1/1 -> Sum2/2, Mux/1  "qdotc"
  Mux2/1 -> heat flux upwards/1, heat flux downwards/1
  Bus Selector/2 -> Mux3/2  "<Tr>"
  Ts/1 -> Mux2/1, Mux3/1, ps_s_l/1, Sum/1  "Ts"
  Mux/1 -> wallsurface/1
  Product/1 -> Mux/2, Sum2/3  "qdotr"
  emission_in/1 -> view_factor/1
  Bus Selector/1 -> x2RelHum_UIBK/1, ps_l/1, Mux2/2, Sum/2  "<Tc>"
  AIB/1 -> Bus Selector/1
  Sum2/1 -> qdots/1
  Mux4/1 -> "[S]"/1
  sigma/1 -> emission_in/1
  Mux3/1 -> Fcn1/1
  Fcn1/1 -> Product/2
  x2RelHum_UIBK/1 -> Gain2/1
  Bus Selector/3 -> x2RelHum_UIBK/2  "<p>"
  Bus Selector/4 -> x2RelHum_UIBK/3  "<x_H2O>"
  Gain2/1 -> phi_i_1/100/1, Product2/1
  lewis/1 -> wallsurface1/1
  ps_l/1 -> Product2/2
  ps_s_l/1 -> Product3/2
  Product3/1 -> Add/1
  Product2/1 -> Add/2
  phis/1 -> Switch/2, Product3/1
  view_factor/1 -> Product/1
  wallsurface1/1 -> Switch/1
  Switch/1 -> Mux4/3
  nomassflow/1 -> Switch/3
  Constant5/1 -> Mux4/6
  Constant4/1 -> Mux4/4
  Constant3/1 -> Mux4/2
  Sum of Elements/1 -> Mux4/5
  Product4/1 -> lewis/1
  Add/1 -> Product4/2
